simulink model "DFIM_model_for_converter"  (R2023b)
settings: Solver=ode45  StartTime=0.0  StopTime=5  FixedStep=5e-6  RelTol=1e-5
InitFcn:
  | run('Maschinen_Parameter_Two.m')
values from neighbouring files (symbols this model uses):
  f = 60    [DefaultSimscapeValues.m]    (also in Newabccoordparam.m = 50)
  Fs = Vs*sqrt(2/3)/(2*pi*f)    [DefaultSimscapeValues.m]    (also in Newabccoordparam.m)
  fsw = 4e3    (= 4000)    [Newabccoordparam.m]
  J = 1.662    [DefaultSimscapeValues.m]    (also in Newabccoordparam.m = 127)
  ki_id = (wni^2)*Lr*sigma    (= 491.599501999)    [Newabccoordparam.m]
  ki_iq = ki_id    (= 491.599501999)    [Newabccoordparam.m]
  ki_n = ((wnn^2)*J)/p    (= 25400)    [Newabccoordparam.m]
  kp_id = (2*wni*sigma*Lr)-Rr    (= 0.5771)    [Newabccoordparam.m]
  kp_iq = kp_id    (= 0.5771)    [Newabccoordparam.m]
  kp_n = (2*wnn*J)/p    (= 2540)    [Newabccoordparam.m]
  Lm = 13.08/377    (= 0.0346949602122)    [DefaultSimscapeValues.m]    (also in Newabccoordparam.m = 0.0025)
  Lr = Lm + Lsi    (= 0.0354960212202)    [DefaultSimscapeValues.m]    (also in Newabccoordparam.m = 0.002587)
  Ls = Lm + Lsi    (= 0.0354960212202)    [DefaultSimscapeValues.m]    (also in Newabccoordparam.m = 0.002587)
  p = 2    [DefaultSimscapeValues.m]    (also in Newabccoordparam.m)
  Rr = 0.228    [DefaultSimscapeValues.m]    (also in Newabccoordparam.m = 0.0029)
  Rs = 0.087    [DefaultSimscapeValues.m]    (also in Newabccoordparam.m = 0.0026)
  sigma = 1- Lm^2/(Ls*Lr)    (= 0.0446259584738)    [DefaultSimscapeValues.m]    (also in Newabccoordparam.m = 0.0661284179513)
  Tem = 12732    [Newabccoordparam.m]
  Vbus = Vr_stator*sqrt(2)    [Newabccoordparam.m]
  Vs = 460    [DefaultSimscapeValues.m]    (also in Newabccoordparam.m = 690)
undefined symbols (not defined in the file or in its folder): DiscIntNeverNeededParam
libraries: spsSeriesRLCBranchLib x9, spsdq0toabcLib x3, spsControlledCurrentSourceLib x3, spsControlledVoltageSourceLib x3, spsabctodq0Lib x3, spsGroundLib x3, spsThreePhaseSineGeneratorLib x2, spsThreePhaseVIMeasurementLib x2, spsDCVoltageSourceLib x1, spsPWMGenerator2LevelLib x1, spsThreePhaseProgrammableVoltageSourceLib x1, spsUniversalBridgeLib x1
settings Model: Creator=ferjani  LastModifiedBy=collins

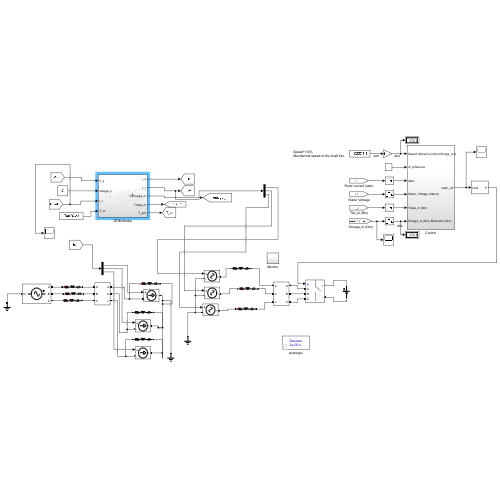
[thumbnail: Simulink's stored preview of the top-level diagram]
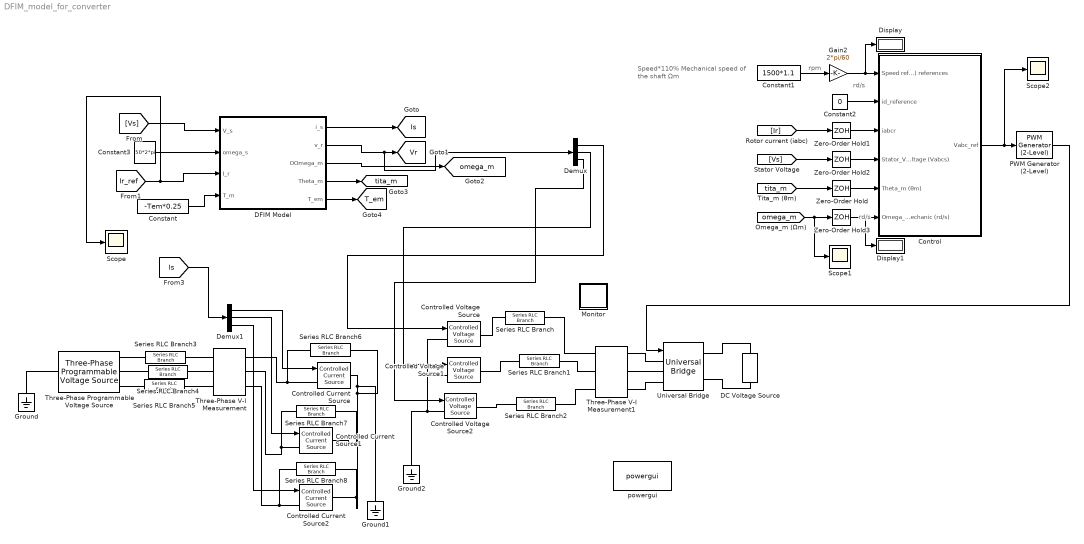
== system DFIM_model_for_converter ==
  note: rd/s
  note: rd/s
  note: Speed*110%
      | Mechanical speed of the shaft Ωm
  note: rpm
  Constant : Constant  Value=-Tem*0.25
  Constant1 : Constant  Value=1500*1.1
  Constant2 : Constant  Value=0
  Constant3 : Constant  Value=50*2*pi
  Control : Subsystem
  Controlled Current Source : spsControlledCurrentSourceLib/Controlled Current Source  Initialize=on  Source_Type=AC  Amplitude=0  Phase=0  Frequency=0  Measurements=None
  Controlled Current Source1 : spsControlledCurrentSourceLib/Controlled Current Source  Initialize=on  Source_Type=AC  Amplitude=0  Phase=0  Frequency=0  Measurements=None
  Controlled Current Source2 : spsControlledCurrentSourceLib/Controlled Current Source  Initialize=on  Source_Type=AC  Amplitude=0  Phase=0  Frequency=0  Measurements=None
  Controlled Voltage Source : spsControlledVoltageSourceLib/Controlled Voltage Source  Initialize=on  Source_Type=AC  Amplitude=0  Phase=0  Frequency=0  Measurements=None
  Controlled Voltage Source1 : spsControlledVoltageSourceLib/Controlled Voltage Source  Initialize=on  Source_Type=AC  Amplitude=0  Phase=0  Frequency=0  Measurements=None
  Controlled Voltage Source2 : spsControlledVoltageSourceLib/Controlled Voltage Source  Initialize=on  Source_Type=AC  Amplitude=0  Phase=0  Frequency=0  Measurements=None
  DC Voltage Source : spsDCVoltageSourceLib/DC Voltage Source  Amplitude=Vbus  Measurements=None
  DFIM Model : Subsystem
  Demux : Demux  Outputs=3
  Demux1 : Demux  Outputs=3
  Display : Display
  Display1 : Display
  Gain2 : Gain  Gain=2*pi/60
  Ground : spsGroundLib/Ground  LConnTagsString=a
  Ground1 : spsGroundLib/Ground  LConnTagsString=a
  Ground2 : spsGroundLib/Ground  LConnTagsString=a
  Monitor : Subsystem
  PWM Generator (2-Level) : spsPWMGenerator2LevelLib/PWM Generator (2-Level)  ModulatorType=Three-phase bridge (6 pulses)  ModulatorMode=Unsynchronized  Fc=fsw  Pc=90  nF=27  MinMax="[ -1  1 ]"  SamplingTechnique=Natural  ModulatingSignals=off  m=0.8  Freq=60  Phase=0  Ts=0  ShowCarrierOutport=off
  Scope : Scope
  Scope1 : Scope
  Scope2 : Scope
  Series RLC Branch{,1..5} (6 alike) : spsSeriesRLCBranchLib/Series RLC Branch  LConnTagsString=__new0  RConnTagsString=__new0  BranchType=RLC  Resistance=1e-6  Inductance=0  SetiL0=off  InitialCurrent=0  Capacitance=0  Setx0=off  InitialVoltage=0  Measurements=None
  Series RLC Branch6 : spsSeriesRLCBranchLib/Series RLC Branch  LConnTagsString=__new0  RConnTagsString=__new0  BranchType=RLC  Resistance=1e100  Inductance=0  SetiL0=off  InitialCurrent=0  Capacitance=0  Setx0=off  InitialVoltage=0  Measurements=None
  Series RLC Branch7 : spsSeriesRLCBranchLib/Series RLC Branch  LConnTagsString=__new0  RConnTagsString=__new0  BranchType=RLC  Resistance=1e100  Inductance=0  SetiL0=off  InitialCurrent=0  Capacitance=0  Setx0=off  InitialVoltage=0  Measurements=None
  Series RLC Branch8 : spsSeriesRLCBranchLib/Series RLC Branch  LConnTagsString=__new0  RConnTagsString=__new0  BranchType=RLC  Resistance=1e100  Inductance=0  SetiL0=off  InitialCurrent=0  Capacitance=0  Setx0=off  InitialVoltage=0  Measurements=None
  Three-Phase Programmable Voltage Source : spsThreePhaseProgrammableVoltageSourceLib/Three-Phase Programmable Voltage Source  PositiveSequence="[Vs  0 f]"  VariationEntity=None  VariationType=Table of time-amplitude pairs  VariationTypeAlt=Step  VariationStep=0.5  VariationRate=10  VariationMagnitude=0.3  VariationFrequency=2  VariationTiming=[1 2]  VariationPhaseA=off  Amplitudes=[1 0.8 1.2 1.0]  TimeValues=[0 0.1 0.15 0.2]  HarmonicGeneration=off  HarmonicA=[3 0.2 -25 0]  HarmonicB=[2 0.15 35 2]  Timing="[0.05  3]"  BusType=swing  Pref=0  Qref=0  Qmin=-inf  Qmax=inf
  Three-Phase V-I Measurement : spsThreePhaseVIMeasurementLib/Three-Phase V-I Measurement  VoltageMeasurement=phase-to-ground  SetLabelV=on  LabelV=Vs  Vpu=off  VpuLL=off  CurrentMeasurement=yes  SetLabelI=on  LabelI=Is1  Ipu=off  Pbase=100e6  Vbase=500e3  OutputType=Complex  PhasorSimulation=off  PSBequivalent=0
  Three-Phase V-I Measurement1 : spsThreePhaseVIMeasurementLib/Three-Phase V-I Measurement  VoltageMeasurement=phase-to-phase  SetLabelV=on  LabelV=Vr1  Vpu=off  VpuLL=off  CurrentMeasurement=yes  SetLabelI=on  LabelI=Ir  Ipu=off  Pbase=100e6  Vbase=500e3  OutputType=Complex  PhasorSimulation=off  PSBequivalent=0
  Universal Bridge : spsUniversalBridgeLib/Universal Bridge  Arms=3  SnubberResistance=1e5  SnubberCapacitance=inf  Device=Ideal Switches  Ron=1e-3  Lon=0  ForwardVoltages="[  0  0  ]"  ForwardVoltage=0  GTOparameters=[ 10e-6 , 20e-6 ]  IGBTparameters=[ 1e-6 , 2e-6 ]  Measurements=None  Measurements_2=None  converterType=Rectifier
  Zero-Order Hold{,1..3} (4 alike) : ZeroOrderHold  SampleTime=1/fsw
  powergui : sps_lib/powergui  Priority=1  SimulationMode=Discrete  SampleTime=5e-5  frequency=60  Iterations=50  frequencyindice=0  Pbase=100e6  ErrMax=1e-4  UnitsV=kV  UnitsW=MW  buscounter=0  FunctionMessages=off  echomessages=off  EnableUseOfTLC=off  CurrentSourceSwitches=off  DisableSnubberDevices=off  DisableRonSwitches=off  DisableVfSwitches=off  DisplayEquations=off  AutomaticDiscreteSolvers=off  SolverType=Tustin/Backward Euler (TBE)  Interpol=off  ExternalGateDelay=off  methode=off  Ts=100  x0status=blocks  SPID=on  SwTol=0  HookPort=off  NonlinearTolerance=1e-4  nMaxIteration=100  ContinueOnMaxIteration=off  RestoreLinks=warning  ResistiveCurrentMeasurement=off  Frange=[0:2:500]  Ylog=off  Xlog=on  ShowGrid=off  save=off  variable=ZData  structure=0  ZoomFFT=off  StartTime=0.0  cycles=1  DisplayStyle=1  fundamental=60  FreqAxis=off  MaxFrequency=1000  frequencyindicesteady=1  RmsSteady=1  display=off
  tag scope: Is=global, T_em=global, Vr=global, omega_m=global, tita_m=global
  wires:
  DFIM Model/4(Theta_m) -> [tita_m]
  Demux1/2 -> Controlled Current Source1/1
  DFIM Model/5(T_em) -> [T_em]
  Demux1/1 -> Controlled Current Source/1
  Zero-Order Hold1/1 -> Control/3(iabcr)
  Constant2/1 -> Control/2(id_reference)
  Zero-Order Hold3/1 -> Display1/1, Control/6(Omega_m (Ωm) Mechanic (rd/s))
  [Ir] -> Zero-Order Hold1/1
  Constant/1 -> DFIM Model/4(T_m)
  Constant1/1 -> Gain2/1
  [tita_m] -> Zero-Order Hold/1
  Zero-Order Hold/1 -> Control/5(Theta_m (θm))
  Gain2/1 -> Display/1, Control/1(Speed reference (rd/s) Omega_m (Ωm) references)
  [Vs] -> Zero-Order Hold2/1
  Demux/2 -> Controlled Voltage Source1/1
  [omega_m] -> Scope1/1, Zero-Order Hold3/1
  [Is] -> Demux1/1
  Zero-Order Hold2/1 -> Control/4(Stator_Voltage (Vabcs))
  DFIM Model/1(i_s) -> [Is]
  DFIM Model/2(v_r) -> Demux/1, [Vr]
  [Ir_ref] -> Scope/1, DFIM Model/3(I_r)
  Demux/1 -> Controlled Voltage Source/1
  Constant3/1 -> DFIM Model/2(omega_s)
  DFIM Model/3(OOmega_m) -> [omega_m]
  [Vs] -> DFIM Model/1(V_s)
  Demux/3 -> Controlled Voltage Source2/1
  Demux1/3 -> Controlled Current Source2/1
  Control/1(Vabc_ref) -> Scope2/1, PWM Generator (2-Level)/1
  PWM Generator (2-Level)/1 -> Universal Bridge/1
  connections:
  Ground1/LConn1 -- Series RLC Branch6/RConn1 -- Series RLC Branch8/RConn1 -- Controlled Current Source2/RConn1 -- Series RLC Branch7/RConn1 -- Controlled Current Source1/RConn1 -- Controlled Current Source/RConn1
  Three-Phase Programmable Voltage Source/LConn1 -- Ground/LConn1
  Three-Phase V-I Measurement/RConn3 -- Series RLC Branch8/LConn1 -- Controlled Current Source2/LConn1
  Three-Phase V-I Measurement/RConn2 -- Series RLC Branch7/LConn1 -- Controlled Current Source1/LConn1
  Three-Phase Programmable Voltage Source/RConn3 -- Series RLC Branch5/LConn1
  Series RLC Branch3/LConn1 -- Three-Phase Programmable Voltage Source/RConn1
  Series RLC Branch4/RConn1 -- Three-Phase V-I Measurement/LConn2
  Three-Phase V-I Measurement/RConn1 -- Series RLC Branch6/LConn1 -- Controlled Current Source/LConn1
  Ground2/LConn1 -- Controlled Voltage Source1/LConn1 -- Controlled Voltage Source/LConn1 -- Controlled Voltage Source2/LConn1
  Universal Bridge/RConn1 -- DC Voltage Source/RConn1
  Universal Bridge/RConn2 -- DC Voltage Source/LConn1
  Three-Phase V-I Measurement1/LConn1 -- Universal Bridge/LConn1
  Three-Phase V-I Measurement1/LConn2 -- Universal Bridge/LConn2
  Three-Phase V-I Measurement1/LConn3 -- Universal Bridge/LConn3
  Controlled Voltage Source/RConn1 -- Series RLC Branch/LConn1
  Series RLC Branch/RConn1 -- Three-Phase V-I Measurement1/RConn1
  Controlled Voltage Source1/RConn1 -- Series RLC Branch1/LConn1
  Series RLC Branch1/RConn1 -- Three-Phase V-I Measurement1/RConn2
  Controlled Voltage Source2/RConn1 -- Series RLC Branch2/LConn1
  Series RLC Branch2/RConn1 -- Three-Phase V-I Measurement1/RConn3
  Three-Phase V-I Measurement/LConn1 -- Series RLC Branch3/RConn1
  Three-Phase Programmable Voltage Source/RConn2 -- Series RLC Branch4/LConn1
  Series RLC Branch5/RConn1 -- Three-Phase V-I Measurement/LConn3

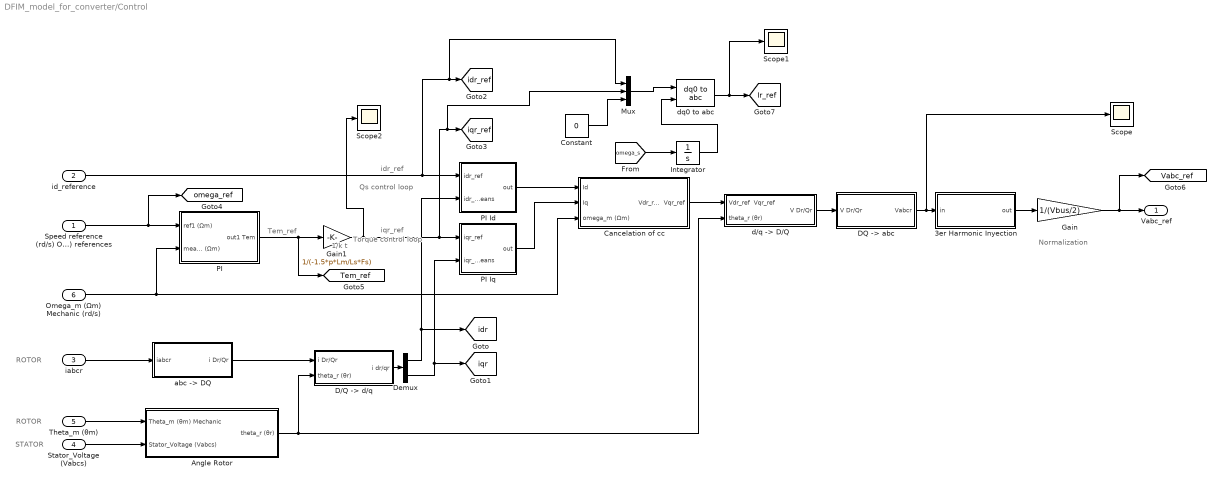
== system DFIM_model_for_converter/Control ==
  note: Normalization
  note: Torque control loop
  note: 1/k t
  note: STATOR
  note: ROTOR
  note: iqr_ref
  note: Tem_ref
  note: idr_ref
  note: ROTOR
  note: Qs control loop
  Speed reference (rd/s) Omega_m (Ωm) references : Inport
  id_reference : Inport  Port=2
  iabcr : Inport  Port=3
  Stator_Voltage (Vabcs) : Inport  Port=4
  Theta_m (θm) : Inport  Port=5
  Omega_m (Ωm) Mechanic (rd/s) : Inport  Port=6
  " Angle Rotor" : Subsystem
  3er Harmonic Inyection : Subsystem
  Cancelation of cc : Subsystem
  Constant : Constant  Value=0
  "D/Q -> d/q" : Subsystem
  "DQ -> abc" : Subsystem
  Demux : Demux  Outputs=2
  Gain : Gain  Gain=1/(Vbus/2)
  Gain1 : Gain  Gain=1/(-1.5*p*Lm/Ls*Fs)
  Integrator : Integrator
  Mux : Mux  Inputs=3
  PI : Subsystem
  PI Id : Subsystem
  PI Iq : Subsystem
  Scope : Scope
  Scope1 : Scope
  Scope2 : Scope
  "abc -> DQ " : Subsystem
  "d/q -> D/Q " : Subsystem
  dq0 to abc : spsdq0toabcLib/dq0 to abc  Alignment=90 degrees behind phase A axis
  Vabc_ref : Outport  VectorParamsAs1DForOutWhenUnconnected=off
  tag scope: Ir_ref=global, Tem_ref=global, Vabc_ref=global, idr=global, idr_ref=global, iqr=global, iqr_ref=global, omega_ref=global
  wires:
  "DQ -> abc"/1(Vabcr) -> Scope/1, 3er Harmonic Inyection/1(in)
  "d/q -> D/Q "/1(V Dr/Qr) -> "DQ -> abc"/1(V Dr/Qr)
  iabcr/1 -> "abc -> DQ "/1(iabcr)
  "abc -> DQ "/1(i Dr/Qr) -> "D/Q -> d/q"/1(i Dr/Qr)
  3er Harmonic Inyection/1(out) -> Gain/1
  Theta_m (θm)/1 -> " Angle Rotor"/1(Theta_m (θm) Mechanic)
  Stator_Voltage (Vabcs)/1 -> " Angle Rotor"/2(Stator_Voltage (Vabcs))
  " Angle Rotor"/1(theta_r (θr)) -> "D/Q -> d/q"/2(theta_r (θr)), "d/q -> D/Q "/2(theta_r (θr))
  PI Id/1(out) -> Cancelation of cc/1(Id)
  PI Iq/1(out) -> Cancelation of cc/2(Iq)
  Omega_m (Ωm) Mechanic (rd/s)/1 -> PI/2("means1 (Ωm) "), Cancelation of cc/3(omega_m (Ωm))
  "D/Q -> d/q"/1(i dr/qr) -> Demux/1
  Demux/2 -> [iqr], PI Iq/2(iqr_means)
  Demux/1 -> [idr], PI Id/2(idr_means)
  PI/1(out1 Tem) -> [Tem_ref], Gain1/1
  Gain1/1 -> Scope2/1, Mux/2, [iqr_ref], PI Iq/1(iqr_ref)
  id_reference/1 -> Mux/1, [idr_ref], PI Id/1(idr_ref)
  Cancelation of cc/1(Vdr_ref  Vqr_ref) -> "d/q -> D/Q "/1(Vdr_ref  Vqr_ref)
  Speed reference (rd/s) Omega_m (Ωm) references/1 -> [omega_ref], PI/1("ref1 (Ωm) ")
  Gain/1 -> [Vabc_ref], Vabc_ref/1
  Constant/1 -> Mux/3
  Mux/1 -> dq0 to abc/1
  [omega_s] -> Integrator/1
  Integrator/1 -> dq0 to abc/2
  dq0 to abc/1 -> Scope1/1, [Ir_ref]

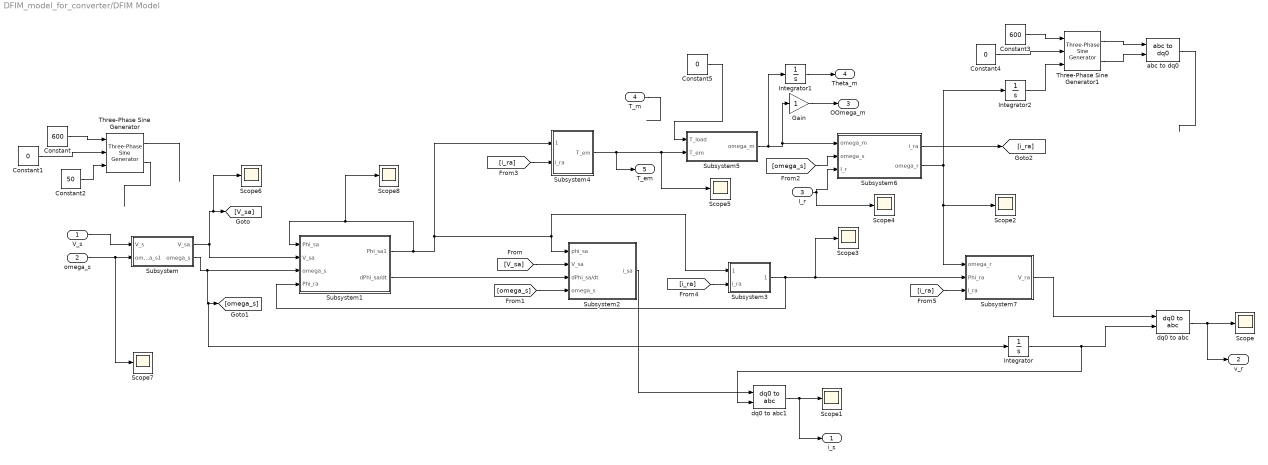
== system DFIM_model_for_converter/DFIM Model ==
  V_s : Inport
  omega_s : Inport  Port=2
  I_r : Inport  Port=3
  T_m : Inport  Port=4
  Constant : Constant  Value=600
  Constant1 : Constant  Value=0
  Constant2 : Constant  Value=50
  Constant3 : Constant  Value=600
  Constant4 : Constant  Value=0
  Constant5 : Constant  Value=0
  Gain : Gain
  Integrator : Integrator
  Integrator1 : Integrator
  Integrator2 : Integrator
  Scope{,1..8} (9 alike) : Scope
  Subsystem : Subsystem
  Subsystem1 : Subsystem
  Subsystem2 : Subsystem
  Subsystem3 : Subsystem
  Subsystem4 : Subsystem
  Subsystem5 : Subsystem
  Subsystem6 : Subsystem
  Subsystem7 : Subsystem
  Three-Phase Sine Generator : spsThreePhaseSineGeneratorLib/Three-Phase Sine Generator  Ts=0
      settings: LibrarySourceBlock=|
      | sps_lib/Sources/Signal Generator Sources/Three-Phase
      | Sine Generator
  Three-Phase Sine Generator1 : spsThreePhaseSineGeneratorLib/Three-Phase Sine Generator  Ts=0
      settings: LibrarySourceBlock=|
      | sps_lib/Sources/Signal Generator Sources/Three-Phase
      | Sine Generator
  abc to dq0 : spsabctodq0Lib/abc to dq0  Alignment=90 degrees behind phase A axis
  dq0 to abc : spsdq0toabcLib/dq0 to abc  Alignment=90 degrees behind phase A axis
  dq0 to abc1 : spsdq0toabcLib/dq0 to abc  Alignment=90 degrees behind phase A axis
  i_s : Outport
  v_r : Outport  Port=2
  OOmega_m : Outport  Port=3
  Theta_m : Outport  Port=4
  T_em : Outport  Port=5
  wires:
  [i_ra] -> Subsystem3/2(i_ra)
  dq0 to abc1/1 -> i_s/1, Scope1/1
  Subsystem4/1(T_em) -> T_em/1, Scope5/1, Subsystem5/2(T_em)
  omega_s/1 -> Scope7/1, Subsystem/2(omega_s1)
  Subsystem1/1(Phi_sa1) -> Scope8/1, Subsystem1/1(Phi_sa), Subsystem4/1(phi_sa), Subsystem3/1(phi_sa), Subsystem2/1(phi_sa)
  Subsystem2/1(i_sa) -> dq0 to abc1/1
  [V_sa] -> Subsystem2/2(V_sa)
  V_s/1 -> Subsystem/1(V_s)
  Subsystem5/1(omega_m) -> Integrator1/1, Gain/1, Subsystem6/1(omega_m)
  Integrator/1 -> dq0 to abc1/2, dq0 to abc/2
  T_m/1 -> ?
  Subsystem3/1(phi_ra) -> Subsystem1/4(Phi_ra), Scope3/1, Subsystem7/2(Phi_ra)
  Integrator1/1 -> Theta_m/1
  I_r/1 -> Subsystem6/3(I_r), Scope4/1
  Subsystem6/1(i_ra) -> [i_ra]
  [i_ra] -> Subsystem7/3(i_ra)
  Gain/1 -> OOmega_m/1
  [omega_s] -> Subsystem6/2(omega_s)
  Subsystem/2(omega_s) -> Integrator/1, [omega_s], Subsystem1/3(omega_s)
  Subsystem1/2(dPhi_sa/dt) -> Subsystem2/3(dPhi_sa/dt)
  Subsystem6/2(omega_r) -> Scope2/1, Subsystem7/1(omega_r), Integrator2/1
  Subsystem7/1(V_ra) -> dq0 to abc/1
  [omega_s] -> Subsystem2/4(omega_s)
  [i_ra] -> Subsystem4/2(i_ra)
  dq0 to abc/1 -> v_r/1, Scope/1
  Constant/1 -> Three-Phase Sine Generator/1
  Constant1/1 -> Three-Phase Sine Generator/2
  Constant2/1 -> Three-Phase Sine Generator/3
  Three-Phase Sine Generator/1 -> ?
  Three-Phase Sine Generator/2 -> ?
  Constant3/1 -> Three-Phase Sine Generator1/1
  Constant4/1 -> Three-Phase Sine Generator1/2
  Integrator2/1 -> Three-Phase Sine Generator1/3
  Three-Phase Sine Generator1/1 -> abc to dq0/1
  Three-Phase Sine Generator1/2 -> abc to dq0/2
  abc to dq0/1 -> ?
  Subsystem/1(V_sa) -> Scope6/1, [V_sa], Subsystem1/2(V_sa)
  Constant5/1 -> Subsystem5/1(T_load)

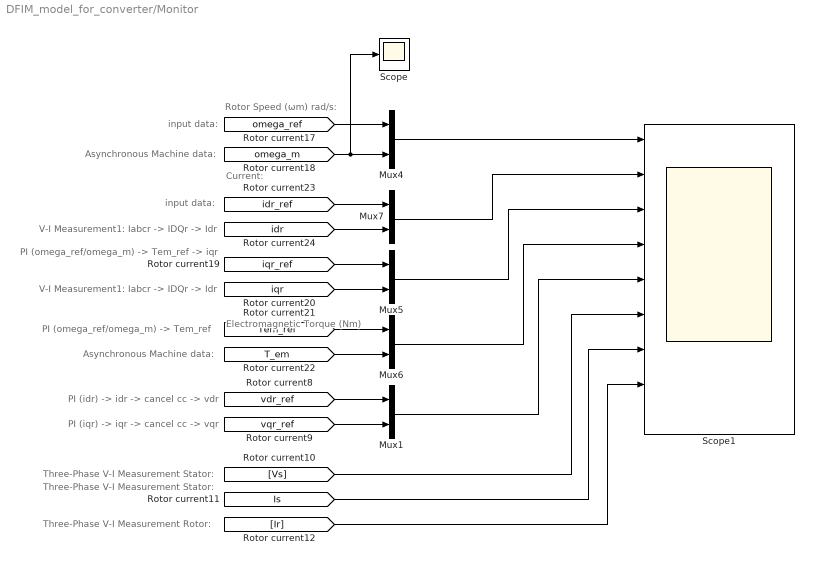
== system DFIM_model_for_converter/Monitor ==
  note: Electromagnetic Torque (Nm)
  note: Three-Phase V-I Measurement Stator:
  note: PI (idr) -> idr -> cancel cc -> vdr
  note: PI (omega_ref/omega_m) -> Tem_ref -> iqr
  note: V-I Measurement1: Iabcr -> IDQr -> Idr
  note: input data:
  note: Current:
  note: Rotor Speed (ωm) rad/s:
  note: Asynchronous Machine data:
  note: input data:
  note: V-I Measurement1: Iabcr -> IDQr -> Idr
  note: PI (omega_ref/omega_m) -> Tem_ref
  note: Asynchronous Machine data:
  note: PI (iqr) -> iqr -> cancel cc -> vqr
  note: Three-Phase V-I Measurement Stator:
  note: Three-Phase V-I Measurement Rotor:
  Mux{1,4..7} (5 alike) : Mux  Inputs=2
  Scope : Scope
  Scope1 : Scope  NumInputPorts=9
  wires:
  [omega_m] -> Scope/1, Mux4/2
  [omega_ref] -> Mux4/1
  [iqr_ref] -> Mux5/1
  [iqr] -> Mux5/2
  [Tem_ref] -> Mux6/1
  [idr] -> Mux7/2
  [idr_ref] -> Mux7/1
  Mux4/1 -> Scope1/1
  [vdr_ref] -> Mux1/1
  [vqr_ref] -> Mux1/2
  Mux7/1 -> Scope1/2
  Mux5/1 -> Scope1/3
  Mux6/1 -> Scope1/4
  Mux1/1 -> Scope1/5
  [Vs] -> Scope1/6
  [Is] -> Scope1/7
  [Ir] -> Scope1/8
  [T_em] -> Mux6/2

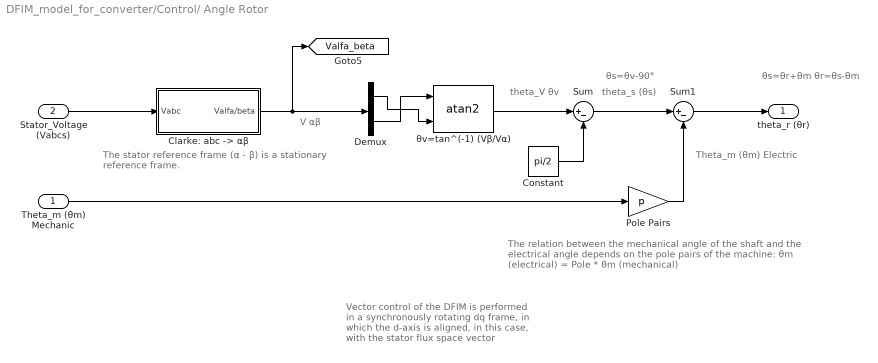
== system DFIM_model_for_converter/Control/ Angle Rotor ==
  note: Theta_m (θm)
      | Electric
  note: theta_V θv
  note: The stator reference frame (α - β) is a stationary
      | reference frame.
  note: The relation between the mechanical angle of the shaft and the
      | electrical angle depends on the pole pairs of the machine:
      |
      | θm (electrical) = Pole * θm (mechanical)
  note: theta_s (θs)
  note: V αβ
  note: θs=θv-90°
  note: θs=θr+θm
      | θr=θs-θm
  note: Vector control of the DFIM is performed in a synchronously rotating dq frame, in which the d-axis is aligned, in this case, with the stator flux space vector
  Theta_m (θm) Mechanic : Inport
  Stator_Voltage (Vabcs) : Inport  Port=2
  "Clarke: abc -> αβ " : Subsystem
  Constant : Constant  Value=pi/2
  Demux : Demux  Outputs=2
  Pole Pairs : Gain  Gain=p
  Sum : Sum  Inputs=|+-
  Sum1 : Sum  Inputs=|+-
  θv=tan^(-1) (Vβ/Vα) : Trigonometry  Operator=atan2
  theta_r (θr) : Outport  VectorParamsAs1DForOutWhenUnconnected=off
  tag scope: Valfa_beta=global
  wires:
  Stator_Voltage (Vabcs)/1 -> "Clarke: abc -> αβ "/1(Vabc)
  Demux/2 -> θv=tan^(-1) (Vβ/Vα)/1
  Demux/1 -> θv=tan^(-1) (Vβ/Vα)/2
  "Clarke: abc -> αβ "/1("Valfa/beta ") -> Demux/1, [Valfa_beta]
  θv=tan^(-1) (Vβ/Vα)/1 -> Sum/1
  Constant/1 -> Sum/2
  Theta_m (θm) Mechanic/1 -> Pole Pairs/1
  Sum/1 -> Sum1/1
  Sum1/1 -> theta_r (θr)/1
  Pole Pairs/1 -> Sum1/2

== system DFIM_model_for_converter/Control/3er Harmonic Inyection ==
  in : Inport
  Gain : Gain  Gain=-0.5
  MinMax : MinMax
  MinMax1 : MinMax  Function=max
  Scope : Scope
  Sum : Sum  Inputs=|++
  Sum1 : Sum  Inputs=|++
  out : Outport  VectorParamsAs1DForOutWhenUnconnected=off
  wires:
  in/1 -> Sum1/1, MinMax1/1, MinMax/1
  MinMax/1 -> Sum/1
  MinMax1/1 -> Sum/2
  Sum1/1 -> out/1
  Sum/1 -> Gain/1
  Gain/1 -> Scope/1, Sum1/2

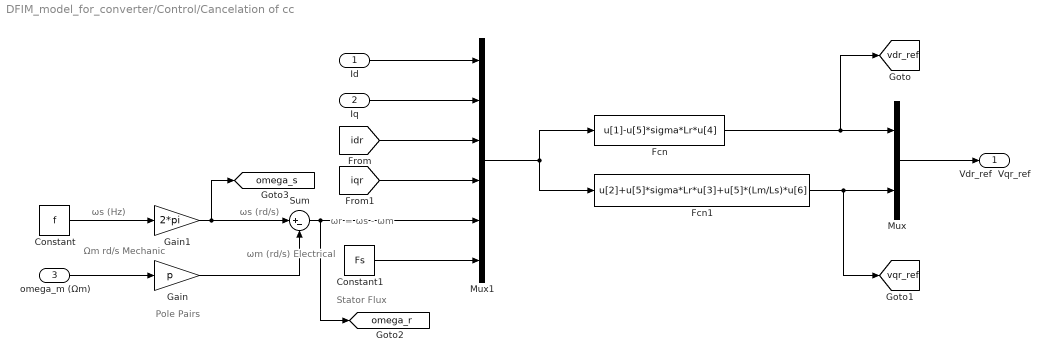
== system DFIM_model_for_converter/Control/Cancelation of cc ==
  note: Stator Flux
  note: Ωm rd/s
      | Mechanic
  note: ωs (Hz)
  note: Pole Pairs
  note: ωr = ωs - ωm
  note: ωs (rd/s)
  note: ωm (rd/s)
      | Electrical
  Id : Inport
  Iq : Inport  Port=2
  omega_m (Ωm) : Inport  Port=3
  Constant : Constant  Value=f
  Constant1 : Constant  Value=Fs
  Fcn : Fcn  Expr=u[1]-u[5]*sigma*Lr*u[4]
  Fcn1 : Fcn  Expr=u[2]+u[5]*sigma*Lr*u[3]+u[5]*(Lm/Ls)*u[6]
  Gain : Gain  Gain=p
  Gain1 : Gain  Gain=2*pi
  Mux : Mux  Inputs=2
  Mux1 : Mux  Inputs=6
  Sum : Sum  Inputs=|+-
  Vdr_ref  Vqr_ref : Outport  VectorParamsAs1DForOutWhenUnconnected=off
  tag scope: omega_r=global, omega_s=global, vdr_ref=global, vqr_ref=global
  wires:
  Mux/1 -> Vdr_ref  Vqr_ref/1
  Fcn/1 -> [vdr_ref], Mux/1
  Fcn1/1 -> [vqr_ref], Mux/2
  Id/1 -> Mux1/1
  Iq/1 -> Mux1/2
  Mux1/1 -> Fcn1/1, Fcn/1
  [idr] -> Mux1/3
  [iqr] -> Mux1/4
  Constant1/1 -> Mux1/6
  omega_m (Ωm)/1 -> Gain/1
  Gain/1 -> Sum/2
  Constant/1 -> Gain1/1
  Gain1/1 -> [omega_s], Sum/1
  Sum/1 -> [omega_r], Mux1/5

== system DFIM_model_for_converter/Control/D//Q -> d//q ==
  i Dr/Qr : Inport
  theta_r (θr) : Inport  Port=2
  Fcn : Fcn  Expr=u(1)*cos(u[3])+u[2]*sin(u[3])
  Fcn1 : Fcn  Expr=-u(1)*sin(u[3])+u[2]*cos(u[3])
  Mux : Mux  Inputs=2
  Mux1 : Mux  Inputs=2
  i dr/qr : Outport  VectorParamsAs1DForOutWhenUnconnected=off
  wires:
  Mux/1 -> i dr/qr/1
  Fcn/1 -> Mux/1
  Fcn1/1 -> Mux/2
  i Dr/Qr/1 -> Mux1/1
  theta_r (θr)/1 -> Mux1/2
  Mux1/1 -> Fcn1/1, Fcn/1

== system DFIM_model_for_converter/Control/DQ -> abc ==
  V Dr/Qr : Inport
  Fcn : Fcn  Expr=u(1)
  Fcn1 : Fcn  Expr=-(u[1]/2)+u[2]*(sqrt(3)/2)
  Fcn2 : Fcn  Expr=-(u[1]/2)-u[2]*(sqrt(3)/2)
  Mux : Mux  Inputs=3
  Vabcr : Outport  VectorParamsAs1DForOutWhenUnconnected=off
  wires:
  Mux/1 -> Vabcr/1
  V Dr/Qr/1 -> Fcn2/1, Fcn1/1, Fcn/1
  Fcn/1 -> Mux/1
  Fcn1/1 -> Mux/2
  Fcn2/1 -> Mux/3

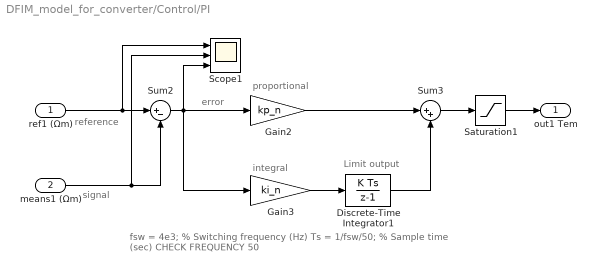
== system DFIM_model_for_converter/Control/PI ==
  note: Limit output
  note: proportional
  note: reference
  note: error
  note: fsw = 4e3;                  % Switching frequency (Hz)
      | Ts = 1/fsw/50;            % Sample time (sec) CHECK FREQUENCY 50
  note: signal
  note: integral
  "ref1 (Ωm) " : Inport
  "means1 (Ωm) " : Inport  Port=2
  Discrete-Time Integrator1 : DiscreteIntegrator  SampleTime=1/fsw  LimitOutput=on  UpperSaturationLimit=Tem  LowerSaturationLimit=-Tem  ICPrevOutput=DiscIntNeverNeededParam  ICPrevScaledInput=DiscIntNeverNeededParam
  Gain2 : Gain  Gain=kp_n
  Gain3 : Gain  Gain=ki_n
  Saturation1 : Saturate  UpperLimit=Tem  LowerLimit=-Tem
  Scope1 : Scope  NumInputPorts=3
  Sum2 : Sum  Inputs=|+-
  Sum3 : Sum  Inputs=|++
  out1 Tem : Outport  VectorParamsAs1DForOutWhenUnconnected=off
  wires:
  Gain2/1 -> Sum3/1
  Sum3/1 -> Saturation1/1
  "ref1 (Ωm) "/1 -> Scope1/1, Sum2/1
  "means1 (Ωm) "/1 -> Scope1/2, Sum2/2
  Sum2/1 -> Scope1/3, Gain3/1, Gain2/1
  Gain3/1 -> Discrete-Time Integrator1/1
  Discrete-Time Integrator1/1 -> Sum3/2
  Saturation1/1 -> out1 Tem/1

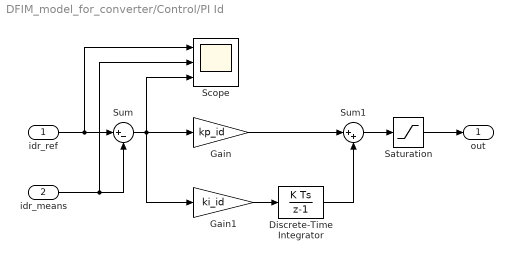
== system DFIM_model_for_converter/Control/PI Id ==
  idr_ref : Inport
  idr_means : Inport  Port=2
  Discrete-Time Integrator : DiscreteIntegrator  SampleTime=1/fsw  LimitOutput=on  UpperSaturationLimit=Vbus/sqrt(3)  LowerSaturationLimit=-Vbus/sqrt(3)  ICPrevOutput=DiscIntNeverNeededParam  ICPrevScaledInput=DiscIntNeverNeededParam
  Gain : Gain  Gain=kp_id
  Gain1 : Gain  Gain=ki_id
  Saturation : Saturate  UpperLimit=Vbus/sqrt(3)  LowerLimit=-Vbus/sqrt(3)
  Scope : Scope  NumInputPorts=3
  Sum : Sum  Inputs=|+-
  Sum1 : Sum  Inputs=|++
  out : Outport  VectorParamsAs1DForOutWhenUnconnected=off
  wires:
  idr_means/1 -> Scope/2, Sum/2
  idr_ref/1 -> Scope/1, Sum/1
  Sum/1 -> Scope/3, Gain1/1, Gain/1
  Gain/1 -> Sum1/1
  Gain1/1 -> Discrete-Time Integrator/1
  Discrete-Time Integrator/1 -> Sum1/2
  Sum1/1 -> Saturation/1
  Saturation/1 -> out/1

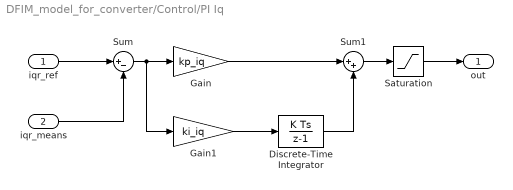
== system DFIM_model_for_converter/Control/PI Iq ==
  iqr_ref : Inport
  iqr_means : Inport  Port=2
  Discrete-Time Integrator : DiscreteIntegrator  SampleTime=1/fsw  LimitOutput=on  UpperSaturationLimit=Vbus/sqrt(3)  LowerSaturationLimit=-Vbus/sqrt(3)  ICPrevOutput=DiscIntNeverNeededParam  ICPrevScaledInput=DiscIntNeverNeededParam
  Gain : Gain  Gain=kp_iq
  Gain1 : Gain  Gain=ki_iq
  Saturation : Saturate  UpperLimit=Vbus/sqrt(3)  LowerLimit=-Vbus/sqrt(3)
  Sum : Sum  Inputs=|+-
  Sum1 : Sum  Inputs=|++
  out : Outport  VectorParamsAs1DForOutWhenUnconnected=off
  wires:
  iqr_means/1 -> Sum/2
  iqr_ref/1 -> Sum/1
  Sum/1 -> Gain1/1, Gain/1
  Gain/1 -> Sum1/1
  Gain1/1 -> Discrete-Time Integrator/1
  Discrete-Time Integrator/1 -> Sum1/2
  Sum1/1 -> Saturation/1
  Saturation/1 -> out/1

== system DFIM_model_for_converter/Control/abc -> DQ  ==
  note: iQr
  note: iDr
  iabcr : Inport
  Fcn : Fcn  Expr=2/3*(u[1]-u[2]/2-u[3]/2)
  Fcn1 : Fcn  Expr=2/3*(u[2]*(sqrt(3)/2)-u[3]*(sqrt(3)/2))
  Mux : Mux  Inputs=2
  i Dr/Qr : Outport  VectorParamsAs1DForOutWhenUnconnected=off
  wires:
  Mux/1 -> i Dr/Qr/1
  iabcr/1 -> Fcn1/1, Fcn/1
  Fcn/1 -> Mux/1
  Fcn1/1 -> Mux/2

== system DFIM_model_for_converter/Control/d//q -> D//Q  ==
  Vdr_ref  Vqr_ref : Inport
  theta_r (θr) : Inport  Port=2
  Fcn : Fcn  Expr=u(1)*cos(u[3])-u[2]*sin(u[3])
  Fcn1 : Fcn  Expr=u(1)*sin(u[3])+u[2]*cos(u[3])
  Mux : Mux  Inputs=2
  Mux1 : Mux  Inputs=2
  V Dr/Qr : Outport  VectorParamsAs1DForOutWhenUnconnected=off
  wires:
  Mux/1 -> V Dr/Qr/1
  Fcn/1 -> Mux/1
  Fcn1/1 -> Mux/2
  Vdr_ref  Vqr_ref/1 -> Mux1/1
  theta_r (θr)/1 -> Mux1/2
  Mux1/1 -> Fcn/1, Fcn1/1

== system DFIM_model_for_converter/DFIM Model/Subsystem ==
  V_s : Inport
  omega_s1 : Inport  Port=2
  Integrator : Integrator
  abc to dq0 : spsabctodq0Lib/abc to dq0  Alignment=90 degrees behind phase A axis
  V_sa : Outport
  omega_s : Outport  Port=2
  wires:
  abc to dq0/1 -> V_sa/1
  V_s/1 -> abc to dq0/1
  Integrator/1 -> abc to dq0/2
  omega_s1/1 -> Integrator/1, omega_s/1

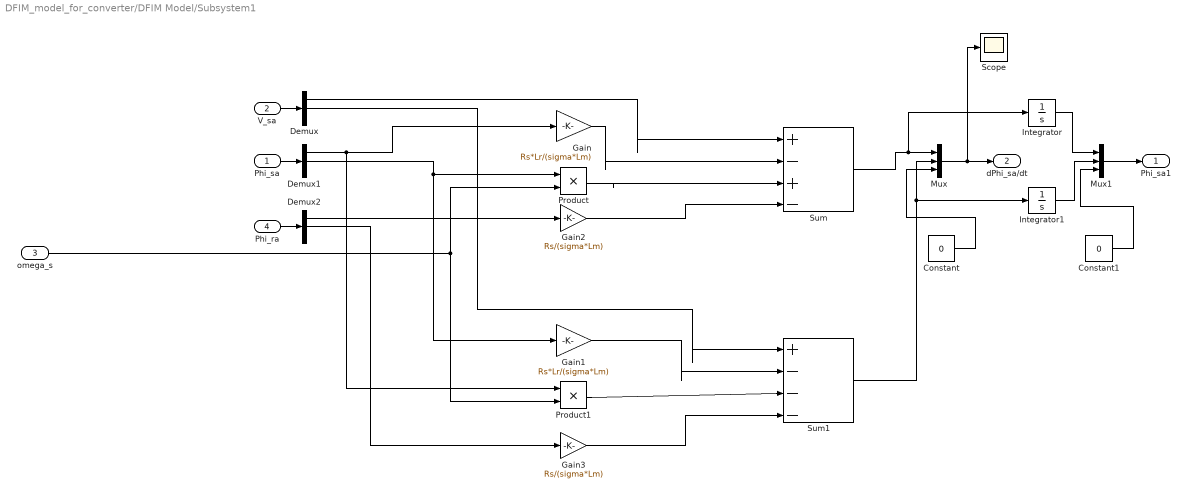
== system DFIM_model_for_converter/DFIM Model/Subsystem1 ==
  Phi_sa : Inport
  V_sa : Inport  Port=2
  omega_s : Inport  Port=3
  Phi_ra : Inport  Port=4
  Constant : Constant  Value=0
  Constant1 : Constant  Value=0
  Demux : Demux  Outputs=3
  Demux1 : Demux  Outputs=3
  Demux2 : Demux  Outputs=3
  Gain : Gain  Gain=Rs*Lr/(sigma*Lm)
  Gain1 : Gain  Gain=Rs*Lr/(sigma*Lm)
  Gain2 : Gain  Gain=Rs/(sigma*Lm)
  Gain3 : Gain  Gain=Rs/(sigma*Lm)
  Integrator : Integrator
  Integrator1 : Integrator
  Mux : Mux  Inputs=3
  Mux1 : Mux  Inputs=3
  Product : Product
  Product1 : Product
  Scope : Scope
  Sum : Sum  Inputs=|+-+-
  Sum1 : Sum  Inputs=|+---
  Phi_sa1 : Outport
  dPhi_sa/dt : Outport  Port=2
  wires:
  Gain/1 -> Sum/2
  Gain2/1 -> Sum/4
  Product/1 -> Sum/3
  Mux/1 -> Scope/1, dPhi_sa/dt/1
  Sum/1 -> Integrator/1, Mux/1
  V_sa/1 -> Demux/1
  Demux/1 -> Sum/1
  Phi_sa/1 -> Demux1/1
  Phi_ra/1 -> Demux2/1
  Gain1/1 -> Sum1/2
  omega_s/1 -> Product/2, Product1/2
  Gain3/1 -> Sum1/4
  Product1/1 -> Sum1/3
  Demux/2 -> Sum1/1
  Sum1/1 -> Integrator1/1, Mux/2
  Integrator/1 -> Mux1/1
  Integrator1/1 -> Mux1/2
  Mux1/1 -> Phi_sa1/1
  Constant/1 -> Mux/3
  Constant1/1 -> Mux1/3
  Demux1/1 -> Product1/1, Gain/1
  Demux2/1 -> Gain2/1
  Demux1/2 -> Product/1, Gain1/1
  Demux2/2 -> Gain3/1

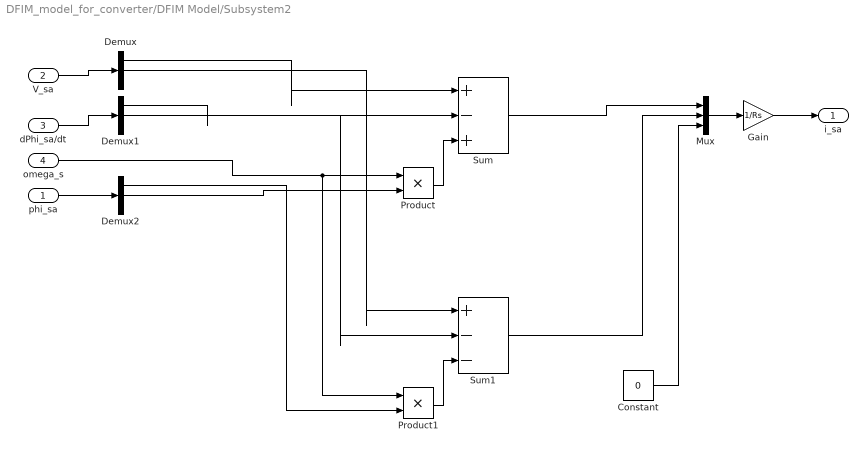
== system DFIM_model_for_converter/DFIM Model/Subsystem2 ==
  phi_sa : Inport
  V_sa : Inport  Port=2
  dPhi_sa/dt : Inport  Port=3
  omega_s : Inport  Port=4
  Constant : Constant  Value=0
  Demux : Demux  Outputs=3
  Demux1 : Demux  Outputs=3
  Demux2 : Demux  Outputs=3
  Gain : Gain  Gain=1/Rs
  Mux : Mux  Inputs=3
  Product : Product
  Product1 : Product
  Sum : Sum  Inputs=|+-+
  Sum1 : Sum  Inputs=|+--
  i_sa : Outport
  wires:
  Product/1 -> Sum/3
  Gain/1 -> i_sa/1
  Mux/1 -> Gain/1
  Constant/1 -> Mux/3
  V_sa/1 -> Demux/1
  Demux/1 -> Sum/1
  dPhi_sa/dt/1 -> Demux1/1
  Demux1/1 -> Sum/2
  omega_s/1 -> Product1/1, Product/1
  phi_sa/1 -> Demux2/1
  Demux2/2 -> Product/2
  Product1/1 -> Sum1/3
  Sum/1 -> Mux/1
  Sum1/1 -> Mux/2
  Demux/2 -> Sum1/1
  Demux1/2 -> Sum1/2
  Demux2/1 -> Product1/2

== system DFIM_model_for_converter/DFIM Model/Subsystem3 ==
  phi_sa : Inport
  i_ra : Inport  Port=2
  Gain : Gain  Gain=Lm/Ls
  Gain1 : Gain  Gain=Lr
  Gain2 : Gain  Gain=Lm*Lm/Ls
  Sum : Sum  Inputs=|++-  RndMeth=Round
  phi_ra : Outport
  wires:
  i_ra/1 -> Gain2/1, Gain1/1
  Sum/1 -> phi_ra/1
  phi_sa/1 -> Gain/1
  Gain/1 -> Sum/1
  Gain1/1 -> Sum/2
  Gain2/1 -> Sum/3

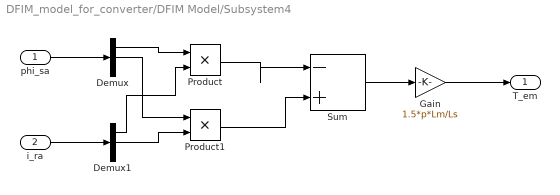
== system DFIM_model_for_converter/DFIM Model/Subsystem4 ==
  phi_sa : Inport
  i_ra : Inport  Port=2
  Demux : Demux  Outputs=3
  Demux1 : Demux  Outputs=3
  Gain : Gain  Gain=1.5*p*Lm/Ls
  Product : Product
  Product1 : Product
  Sum : Sum  Inputs=|-+
  T_em : Outport
  wires:
  Gain/1 -> T_em/1
  Product1/1 -> Sum/2
  Sum/1 -> Gain/1
  i_ra/1 -> Demux1/1
  Demux1/1 -> Product/2
  phi_sa/1 -> Demux/1
  Product/1 -> Sum/1
  Demux/1 -> Product/1
  Demux/2 -> Product1/1
  Demux1/2 -> Product1/2

== system DFIM_model_for_converter/DFIM Model/Subsystem5 ==
  T_load : Inport
  T_em : Inport  Port=2
  Gain : Gain  Gain=1/(J*p)
  Integrator : Integrator
  Scope : Scope
  Sum : Sum  Inputs=|+-
  omega_m : Outport
  wires:
  Sum/1 -> Gain/1
  T_load/1 -> Sum/2
  T_em/1 -> Sum/1
  Gain/1 -> Integrator/1
  Integrator/1 -> Scope/1, omega_m/1

== system DFIM_model_for_converter/DFIM Model/Subsystem6 ==
  omega_m : Inport
  omega_s : Inport  Port=2
  I_r : Inport  Port=3
  Integrator : Integrator
  Scope : Scope
  Sum : Sum  Inputs=|+-
  abc to dq0 : spsabctodq0Lib/abc to dq0  Alignment=90 degrees behind phase A axis
  i_ra : Outport
  omega_r : Outport  Port=2
  wires:
  omega_m/1 -> Sum/2
  Sum/1 -> Integrator/1, omega_r/1
  omega_s/1 -> Sum/1
  I_r/1 -> abc to dq0/1
  abc to dq0/1 -> Scope/1, i_ra/1
  Integrator/1 -> abc to dq0/2

== system DFIM_model_for_converter/DFIM Model/Subsystem7 ==
  omega_r : Inport
  Phi_ra : Inport  Port=2
  i_ra : Inport  Port=3
  Derivative : Derivative
  Gain : Gain  Gain=Rr
  Product : Product
  Scope : Scope
  Sum : Sum  Inputs=|+++
  V_ra : Outport
  wires:
  Product/1 -> Sum/1
  Phi_ra/1 -> Product/2, Derivative/1
  omega_r/1 -> Product/1
  Gain/1 -> Sum/3
  Sum/1 -> Scope/1, V_ra/1
  Derivative/1 -> Sum/2
  i_ra/1 -> Gain/1

== system DFIM_model_for_converter/Control/ Angle Rotor/Clarke: abc -> αβ  ==
  Vabc : Inport
  Fcn : Fcn  Expr=2/3*(u[1]-u[2]/2-u[3]/2)
  Fcn1 : Fcn  Expr=2/3*(u[2]*(sqrt(3)/2)-u[3]*(sqrt(3)/2))
  Mux : Mux  Inputs=2
  "Valfa/beta " : Outport  VectorParamsAs1DForOutWhenUnconnected=off
  wires:
  Mux/1 -> "Valfa/beta "/1
  Vabc/1 -> Fcn1/1, Fcn/1
  Fcn/1 -> Mux/1
  Fcn1/1 -> Mux/2
